simulink model "t"  (R2019a)
settings: Solver=VariableStepAuto  StartTime=0.0  StopTime=100  RelTol=1e-3
undefined symbols (not defined in the file): A, B, C, E, F
settings Model: Creator=julia  LastModifiedBy=julia

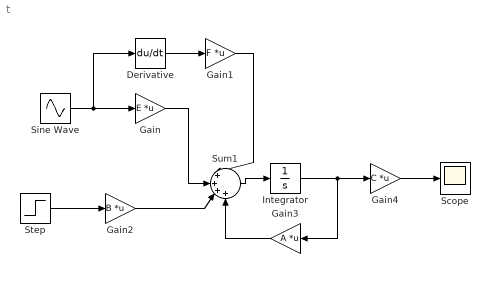
== system t ==
  Derivative : Derivative
  Gain : Gain  Gain=E  Multiplication=Matrix(K*u)
  Gain1 : Gain  Gain=F  Multiplication=Matrix(K*u)
  Gain2 : Gain  Gain=B  Multiplication=Matrix(K*u)
  Gain3 : Gain  Gain=A  Multiplication=Matrix(K*u)
  Gain4 : Gain  Gain=C  Multiplication=Matrix(K*u)
  Integrator : Integrator
  Scope : Scope
  Sine Wave : Sin  Amplitude=0.1  Frequency=pi  SampleTime=0
  Step : Step  SampleTime=0
  Sum1 : Sum  Inputs=|++++
  wires:
  Sine Wave/1 -> Derivative/1, Gain/1
  Derivative/1 -> Gain1/1
  Step/1 -> Gain2/1
  Integrator/1 -> Gain4/1, Gain3/1
  Sum1/1 -> Integrator/1
  Gain4/1 -> Scope/1
  Gain2/1 -> Sum1/3
  Gain3/1 -> Sum1/4
  Gain/1 -> Sum1/2
  Gain1/1 -> Sum1/1
